simulink model "noise_lti_psd"  (R2015a)
settings: Solver=ode45  StartTime=0.0  StopTime=Tsim  RelTol=1e-3
undefined symbols (not defined in the file or in its folder): ts
libraries: simulink_extras x4, commnoisgen2 x2
settings Model: Creator=mainster  LastModifiedBy=mainster

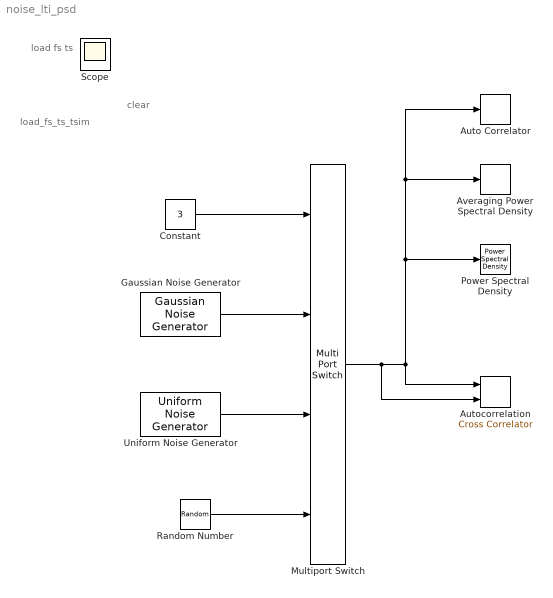
== system noise_lti_psd ==
  note: clear
  note: load_fs_ts_tsim
  note: load fs ts
  Auto Correlator : simulink_extras/Additional Sinks/Auto Correlator  npts=100  HowOften=50  sampleT=0.1
  "Autocorrelation " : simulink_extras/Additional Sinks/Cross Correlator  npts=1e3  HowOften=500  sampleT=ts
  Averaging Power Spectral Density : simulink_extras/Additional Sinks/Averaging Power Spectral Density  npts=128  fftpts=512  HowOften=64  sampleT=ts
  Constant : Constant  Value=3
  Gaussian Noise Generator : commnoisgen2/Gaussian Noise Generator  m=0  d=1  s=41  Ts=ts  frameBased=off  sampPerFrame=1  orient=off  outDataType=double
  Multiport Switch : MultiPortSwitch
  Power Spectral Density : simulink_extras/Additional Sinks/Power Spectral Density  npts=1280  fftpts=5120  HowOften=64*8  sampleT=ts
  Random Number : RandomNumber  SampleTime=ts
  Uniform Noise Generator : commnoisgen2/Uniform Noise Generator  low=0  up=1  seed=31  Ts=ts  frameBased=off  sampPerFrame=1  orient=off  outDataType=double
  Scope : Scope
      settings: ShowLegends=on  TimeRange=0.005  YMin=-1  YMax=1  ScrollMode=on
  wires:
  Constant/1 -> Multiport Switch/1
  Gaussian Noise Generator/1 -> Multiport Switch/2
  Uniform Noise Generator/1 -> Multiport Switch/3
  Random Number/1 -> Multiport Switch/4
  Multiport Switch/1 -> "Autocorrelation "/2, Auto Correlator/1, Averaging Power Spectral Density/1, Power Spectral Density/1, "Autocorrelation "/1
